simulink model "simActuatorPositionControl"  (R2022a)
settings: Solver=VariableStepAuto  StartTime=0.0  StopTime=10  FixedStep=0.001  MaxStep=0.01  RelTol=1e-3
InitFcn:
  | addpath('SCADA');
  | initFcn_SCADA;
model workspace (MAT data in the model file):
  WECmotionOnOff = Simulink.Parameter
  WECmotionOnOff.Value = 1
  WECmotionOnOff.DataType = 'auto'
  WECmotionOnOff.Complexity = 'real'
  WECmotionOnOff.Dimensions = [1 1]
values from neighbouring files (symbols this model uses):
  s = scatter(X(iVar),Y(iVar),100,[color(N-i+1,:)])    [postprocess_datafiles_accum_wRV.m]
undefined symbols (not defined in the file or in its folder): g, HIL_act_A_cap, HIL_act_A_rod, HIL_H1T_kd, HIL_H1T_ki, HIL_H1T_kp, HIL_H1T_P1fBias, HIL_H1T_P1negCutIn, HIL_H1T_P1posCutIn, HIL_H1T_P2fBias, HIL_H1T_P2negCutIn, HIL_H1T_P2posCutIn, HIL_scale_sys, HIL_WECpump_A_cap, HIL_WECpump_A_rod, HIL_WECpump_ang2lin, HIL_WECpump_negativeCtrlLimit, HIL_WECpump_negativeLimit, HIL_WECpump_positiveCtrlLimit, HIL_WECpump_positiveLimit, rho, wave_phi, wave_S_w, WEC_A_rad, WEC_B_rad, WEC_dw, WEC_F_amp, WEC_h, WEC_I, WEC_I_inf, WEC_ICs, WEC_L_cm, WEC_L_flap, WEC_m, WEC_phi_e, WEC_T, WEC_W, WEC_w
libraries: fl_lib x24, sh_lib x22, nesl_utility x11, slpidlib x1, simulink x1
(part 1 of 2)
settings Model: TunableVars=motionOnOff  TunableVarsStorageClass=ExportedGlobal  Creator=simmo536  LastModifiedBy=simmo536
settings SolverCC: ZeroCrossAlgorithm=Adaptive
settings OptimizationCC: DefaultParameterBehavior=Inlined
settings DebuggingCC: IgnoredZcDiagnostic=none
settings RTWCC: Toolchain=Microsoft Visual C++ 2019 v16.0 | nmake (64-bit Windows)

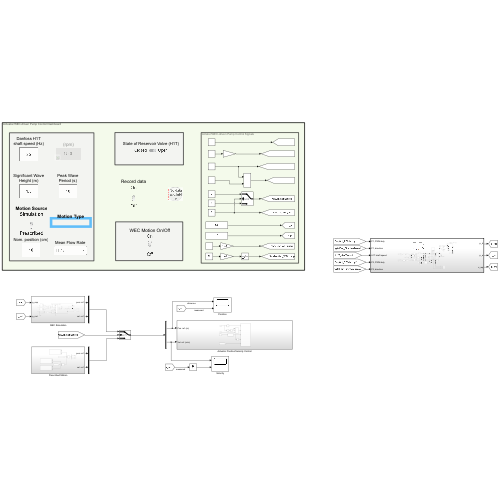
[thumbnail: Simulink's stored preview of the top-level diagram]
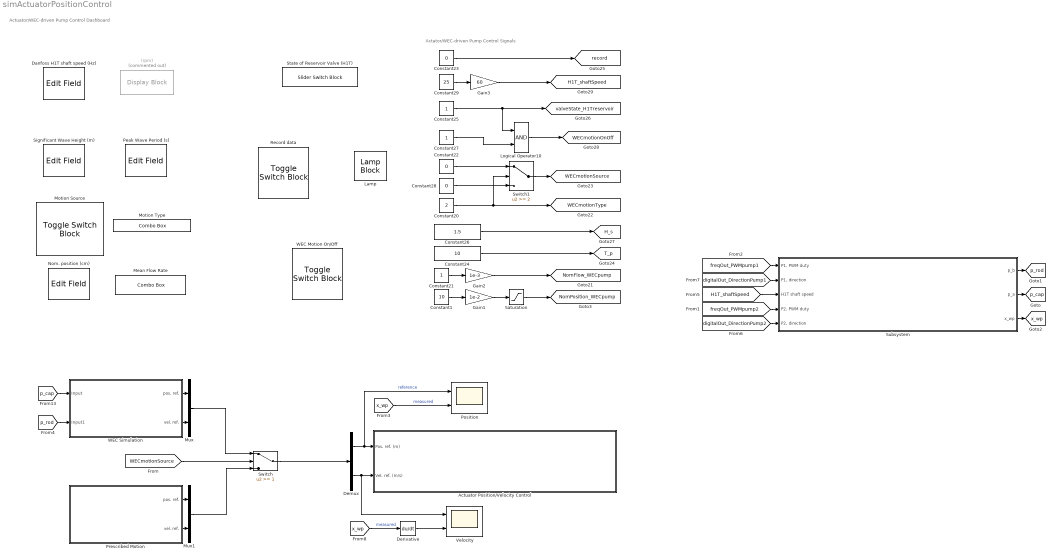
== system simActuatorPositionControl ==
  note: Actator/WEC-driven Pump Control Signals
  note: Actuator/WEC-driven Pump Control Dashboard
  (rpm) : DisplayBlock  Commented=on  LabelPosition=Hide  Format=long  Transparency=1
  Actuator Position/Velocity Control : Subsystem
  Constant1 : Constant  Value=10
  Constant20 : Constant  Value=2
  Constant21 : Constant
  Constant22 : Constant  Value=0
  Constant23 : Constant  Value=0
  Constant24 : Constant  Value=10
  Constant25 : Constant
  Constant26 : Constant  Value=1.5
  Constant27 : Constant
  Constant28 : Constant  Value=0
  Constant29 : Constant  Value=25
  Danfoss H1T shaft speed (Hz) : EditField  LabelPosition=Hide  ShowInitialText=on  Alignment=Center
  Demux : Demux  Outputs=2
  Derivative : Derivative
  Gain1 : Gain  Gain=1e-2
  Gain2 : Gain  Gain=1e-3
  Gain3 : Gain  Gain=60
  Lamp : LampBlock  LabelPosition=Hide
  Logical Operator10 : Logic  AllPortsSameDT=off  OutDataTypeStr=boolean
  Mean Flow Rate : ComboBox  LabelPosition=Hide  SelectedLabel=1 L/s
      settings: Values={{'0 L/s', '1 L/s', '2 L/2'}, [0 1 2]}
  Motion Source : ToggleSwitchBlock  LabelPosition=Hide
      settings: Values={{'Prescribed', 'Simulation'}, [0 1]}
  Motion Type : ComboBox  LabelPosition=Hide  SelectedLabel=Regular Waves
      settings: Values={{'Flow, Constant', 'Regular Waves', 'Irregular Waves', 'Position, Constant'}, [0 2 3 1]}
  Mux : Mux  Inputs=2
  Mux1 : Mux  Inputs=2
  Nom. position (cm) : EditField  LabelPosition=Hide  ShowInitialText=on  Alignment=Center
  Peak Wave Period (s) : EditField  LabelPosition=Hide  ShowInitialText=on  Alignment=Center
  Position : Scope  NumInputPorts=2
  Prescribed Motion : Subsystem
  Record data : ToggleSwitchBlock  LabelPosition=Hide
      settings: Values={{'Off', 'On'}, [0 1]}
  Saturation : Saturate
  Significant Wave Height (m) : EditField  LabelPosition=Hide  ShowInitialText=on  Alignment=Center
  State of Reservoir Valve (H1T) : SliderSwitchBlock  LabelPosition=Hide
      settings: Values={{'Closed', 'Open'}, [0 1]}
  Subsystem : Subsystem  TreatAsAtomicUnit=on
  Switch : Switch  Threshold=1  SaturateOnIntegerOverflow=off  InputSameDT=off
  Switch1 : Switch  Threshold=2  SaturateOnIntegerOverflow=off  InputSameDT=off
  Velocity : Scope  NumInputPorts=2
  WEC Motion On/Off : ToggleSwitchBlock  LabelPosition=Hide
      settings: Values={{'Off', 'On'}, [0 1]}
  WEC Simulation : Subsystem
  tag scope: H1T_shaftSpeed=global, H_s=global, NomFlow_WECpump=global, NomPosition_WECpump=global, T_p=global, WECmotionOnOff=global, WECmotionSource=global, WECmotionType=global, p_cap=global, p_rod=global, record=global, valveState_H1Treservoir=global, x_wp=global
  wires:
  [WECmotionSource] -> Switch/2
  Switch/1 -> Demux/1
  Demux/2 -> Velocity/1, Actuator Position/Velocity Control/2(Vel. ref. (m/s))
  Demux/1 -> Position/1, Actuator Position/Velocity Control/1(Pos. ref. (m))  "reference"
  Constant21/1 -> Gain2/1
  Constant29/1 -> Gain3/1
  Constant28/1 -> Switch1/3
  Gain3/1 -> [H1T_shaftSpeed]
  Switch1/1 -> [WECmotionSource]
  Constant20/1 -> Switch1/2, [WECmotionType]
  Logical Operator10/1 -> [WECmotionOnOff]
  Constant23/1 -> [record]
  Constant22/1 -> Switch1/1
  Constant25/1 -> Logical Operator10/1, [valveState_H1Treservoir]
  Constant26/1 -> [H_s]
  Constant24/1 -> [T_p]
  Gain2/1 -> [NomFlow_WECpump]
  [x_wp] -> Position/2  "measured"
  Constant27/1 -> Logical Operator10/2
  [p_cap] -> WEC Simulation/1(Input)
  WEC Simulation/1(pos. ref.) -> Mux/1
  [p_rod] -> WEC Simulation/2(Input1)
  WEC Simulation/2(vel. ref.) -> Mux/2
  Mux/1 -> Switch/1
  Prescribed Motion/2(vel. ref.) -> Mux1/2
  Mux1/1 -> Switch/3
  Prescribed Motion/1(pos. ref.) -> Mux1/1
  [freqOut_PWMpump1] -> Subsystem/1("P1, PWM duty")
  [digitalOut_DirectionPump1] -> Subsystem/2("P1, direction")
  [H1T_shaftSpeed] -> Subsystem/3(H1T shaft speed)
  [freqOut_PWMpump2] -> Subsystem/4("P2, PWM duty")
  [digitalOut_DirectionPump2] -> Subsystem/5("P2, direction")
  Subsystem/1(p_b) -> [p_rod]
  Subsystem/2(p_a) -> [p_cap]
  Subsystem/3(x_wp) -> [x_wp]
  Derivative/1 -> Velocity/2
  [x_wp] -> Derivative/1  "measured"
  Gain1/1 -> Saturation/1
  Constant1/1 -> Gain1/1
  Saturation/1 -> [NomPosition_WECpump]

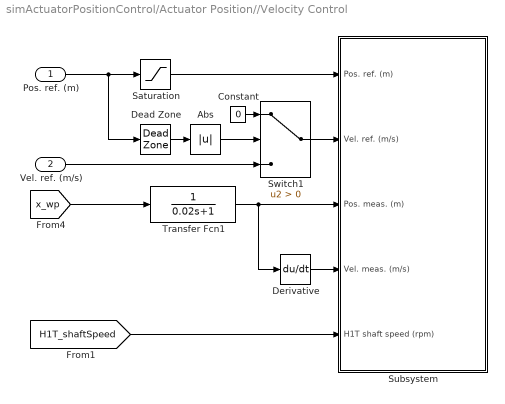
== system simActuatorPositionControl/Actuator Position//Velocity Control ==
  Pos. ref. (m) : Inport
  Vel. ref. (m/s) : Inport  Port=2
  Abs : Abs  SaturateOnIntegerOverflow=off
  Constant : Constant  Value=0
  Dead Zone : DeadZone  LowerValue=HIL_WECpump_negativeCtrlLimit  UpperValue=HIL_WECpump_positiveCtrlLimit
  Derivative : Derivative
  Saturation : Saturate  UpperLimit=HIL_WECpump_positiveCtrlLimit  LowerLimit=HIL_WECpump_negativeCtrlLimit
  Subsystem : Subsystem
  Switch1 : Switch  Criteria=u2 > Threshold  SaturateOnIntegerOverflow=off  InputSameDT=off
  Transfer Fcn1 : TransferFcn  Denominator=[0.02 1]
  wires:
  [x_wp] -> Transfer Fcn1/1
  Pos. ref. (m)/1 -> Saturation/1, Dead Zone/1
  Derivative/1 -> Subsystem/4(Vel. meas. (m/s))
  [H1T_shaftSpeed] -> Subsystem/5(H1T shaft speed (rpm))
  Transfer Fcn1/1 -> Subsystem/3(Pos. meas. (m)), Derivative/1
  Saturation/1 -> Subsystem/1(Pos. ref. (m))
  Dead Zone/1 -> Abs/1
  Abs/1 -> Switch1/2
  Constant/1 -> Switch1/1
  Switch1/1 -> Subsystem/2(Vel. ref. (m/s))
  Vel. ref. (m/s)/1 -> Switch1/3

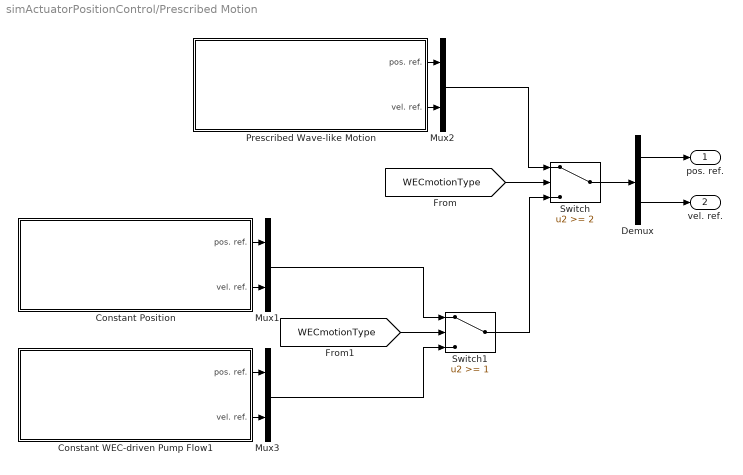
== system simActuatorPositionControl/Prescribed Motion ==
  Constant Position : Subsystem
  Constant WEC-driven Pump Flow1 : Subsystem
  Demux : Demux  Outputs=2
  Mux1 : Mux  Inputs=2
  Mux2 : Mux  Inputs=2
  Mux3 : Mux  Inputs=2
  Prescribed Wave-like Motion : Subsystem
  Switch : Switch  Threshold=2  SaturateOnIntegerOverflow=off  InputSameDT=off
  Switch1 : Switch  Threshold=1  SaturateOnIntegerOverflow=off  InputSameDT=off
  pos. ref. : Outport
  vel. ref. : Outport  Port=2
  wires:
  Prescribed Wave-like Motion/2(vel. ref.) -> Mux2/2
  Prescribed Wave-like Motion/1(pos. ref.) -> Mux2/1
  Mux2/1 -> Switch/1
  Demux/2 -> vel. ref./1
  Demux/1 -> pos. ref./1
  Constant Position/1(pos. ref.) -> Mux1/1
  Constant Position/2(vel. ref.) -> Mux1/2
  [WECmotionType] -> Switch/2
  Switch/1 -> Demux/1
  Constant WEC-driven Pump Flow1/2(vel. ref.) -> Mux3/2
  Constant WEC-driven Pump Flow1/1(pos. ref.) -> Mux3/1
  Mux3/1 -> Switch1/3
  [WECmotionType] -> Switch1/2
  Switch1/1 -> Switch/3
  Mux1/1 -> Switch1/1

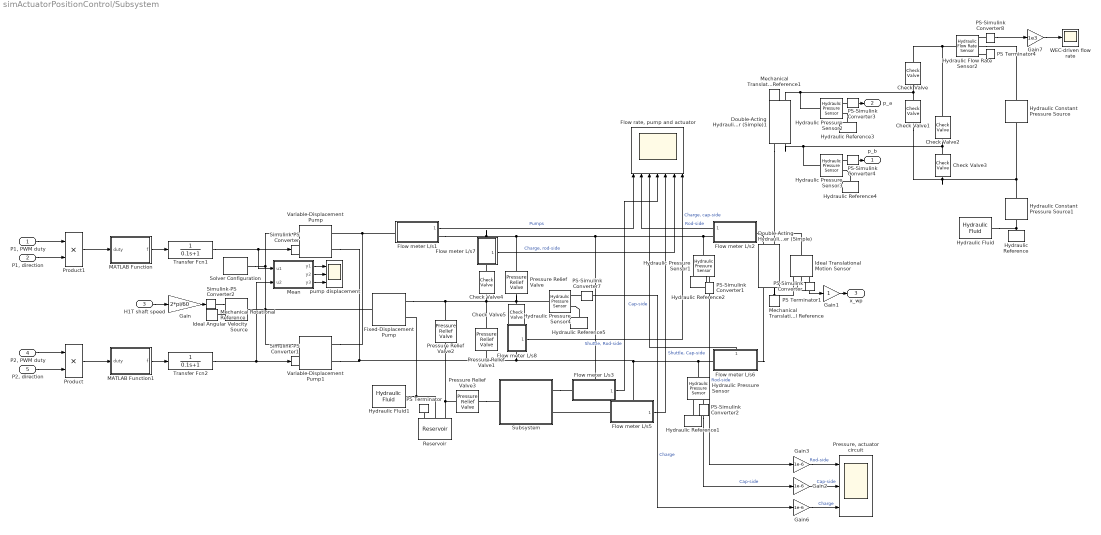
== system simActuatorPositionControl/Subsystem ==
  "P1, PWM duty" : Inport
  "P1, direction" : Inport  Port=2
  H1T shaft speed : Inport  Port=3
  "P2, PWM duty" : Inport  Port=4
  "P2, direction" : Inport  Port=5
  Check Valve{,1..3} (4 alike) : sh_lib/Valves/Directional Valves/Check Valve  area_max=6.1e-4 m^2  pres_crack=10 psi  pres_max=15 psi  C_d=0.7  A_leak=1e-12 m^2  lam_spec=1  B_lam=0.999  Re_cr=12  dynamic=0  tau=0.1 s  area_init=1e-12 m^2
      settings: SourceProductBaseCode=SH  InternalSimscapePortConfiguration="{\"Bottom\":[],\"Left\":[{\"id\":\"A\",\"label\":\"A\",\"type\":\"foundation.hydraulic.hydraulic\"}],\"Right\":[{\"id\":\"B\",\"label\":\"B\",\"type\":\"foundation.hydraulic.hydraulic\"}],\"Top\":[]}"
  Check Valve4 : sh_lib/Valves/Directional Valves/Check Valve  area_max=1e-4 m^2  pres_crack=5 bar  pres_max=6 bar  C_d=0.7  A_leak=1e-12 m^2  lam_spec=1  B_lam=0.999  Re_cr=12  dynamic=0  tau=0.1 s  area_init=1e-12 m^2
      settings: SourceProductBaseCode=SH  InternalSimscapePortConfiguration="{\"Bottom\":[],\"Left\":[{\"id\":\"A\",\"label\":\"A\",\"type\":\"foundation.hydraulic.hydraulic\"}],\"Right\":[{\"id\":\"B\",\"label\":\"B\",\"type\":\"foundation.hydraulic.hydraulic\"}],\"Top\":[]}"
  Check Valve5 : sh_lib/Valves/Directional Valves/Check Valve  area_max=1e-4 m^2  pres_crack=5 bar  pres_max=6 bar  C_d=0.7  A_leak=1e-12 m^2  lam_spec=1  B_lam=0.999  Re_cr=12  dynamic=0  tau=0.1 s  area_init=1e-12 m^2
      settings: SourceProductBaseCode=SH  InternalSimscapePortConfiguration="{\"Bottom\":[],\"Left\":[{\"id\":\"A\",\"label\":\"A\",\"type\":\"foundation.hydraulic.hydraulic\"}],\"Right\":[{\"id\":\"B\",\"label\":\"B\",\"type\":\"foundation.hydraulic.hydraulic\"}],\"Top\":[]}"
  Double-Acting Hydraulic Cylinder (Simple) : sh_lib/Hydraulic Cylinders/Double-Acting Hydraulic Cylinder (Simple)  area_A=HIL_act_A_cap m^2  area_B=HIL_act_A_rod m^2  stroke=1 m  init_pos=0.5 m  penetr_coeff=1e12 N*s/m^2  or=1
      settings: SourceProductBaseCode=SH  InternalSimscapePortConfiguration="{\"Bottom\":[],\"Left\":[{\"id\":\"C\",\"label\":\"C\",\"type\":\"foundation.mechanical.translational.translational\"},{\"id\":\"A\",\"label\":\"A\",\"type\":\"foundation.hydraulic.hydraulic\"}],\"Right\":[{\"id\":\"R\",\"label\":\"R\",\"type\":\"foundation.mechanical.translational.translational\"},{\"id\":\"B\",\"label\":\"B\",\"type\":\"foundation.hydraulic.hydraulic\"}],\"Top\":[]}"
  Double-Acting Hydraulic Cylinder (Simple)1 : sh_lib/Hydraulic Cylinders/Double-Acting Hydraulic Cylinder (Simple)  area_A=HIL_WECpump_A_cap m^2  area_B=HIL_WECpump_A_rod m^2  stroke=HIL_WECpump_positiveLimit - HIL_WECpump_negativeLimit m  init_pos=HIL_WECpump_positiveLimit m  penetr_coeff=1e12 N*s/m^2  or=1
      settings: SourceProductBaseCode=SH  InternalSimscapePortConfiguration="{\"Bottom\":[],\"Left\":[{\"id\":\"C\",\"label\":\"C\",\"type\":\"foundation.mechanical.translational.translational\"},{\"id\":\"A\",\"label\":\"A\",\"type\":\"foundation.hydraulic.hydraulic\"}],\"Right\":[{\"id\":\"R\",\"label\":\"R\",\"type\":\"foundation.mechanical.translational.translational\"},{\"id\":\"B\",\"label\":\"B\",\"type\":\"foundation.hydraulic.hydraulic\"}],\"Top\":[]}"
  Fixed-Displacement Pump : sh_lib/Pumps and Motors/Fixed-Displacement Pump  D=26.7 cm^3/rev  loss_spec=1  w_nominal=188 rad/s  pr_nominal=100e5 Pa  visc_nominal=18 cSt  dens_nominal=900 kg/m^3  efficiency_vol=0.92  no_load_torque=0.05 N*m  torque_pressure_coeff=0.6e-6 N*m/Pa  p_diff_eff_TLU=[100000, 1000000, 2000000] Pa  omega_eff_TLU=[25, 50, 100, 200, 300, 400] rad/s  vol_eff_TLU=[.816, .908, .954, .977, .981, .984; .325, .663, .831, .916, .925, .946; .137, .568, .78, .892, .893, .91]  mech_eff_TLU=[.996, .996, .996, .996, .996, .996; .988, .989, .989, .989, .989, .99; .981, .981, .982, .982, .983, .984]  p_diff_loss_TLU=[100000, 1000000, 2000000] Pa  omega_loss_TLU=[25, 50, 100, 200, 300, 400] rad/s  vol_loss_TLU=[.023, .023, .023, .023, .0285, .032; .0844, .0842, .0845, .084, .1125, .108; .1079, .108, .11, .108, .1605, .18] * 1e-3 m^3/s  mech_loss_TLU=[.002, .002, .002, .002, .002, .002; .0607, .0556, .0556, .0556, .0556, .0505; .1937, .1937, .1833, .1833, .1729, .1626] N*m  pressure_threshold=1e5 Pa  omega_threshold=10 rad/s  quadrant_check=0  pressure_check=0  min_valid_pressure=0 Pa  vol_eff_min=1e-3  vol_eff_max=1  mech_eff_min=1e-3  mech_eff_max=1
      settings: SourceProductBaseCode=SH  InternalSimscapePortConfiguration="{\"Bottom\":[],\"Left\":[{\"id\":\"S\",\"label\":\"S\",\"type\":\"foundation.mechanical.rotational.rotational\"}],\"Right\":[{\"id\":\"P\",\"label\":\"P\",\"type\":\"foundation.hydraulic.hydraulic\"},{\"id\":\"T\",\"label\":\"T\",\"type\":\"foundation.hydraulic.hydraulic\"}],\"Top\":[]}"
  Flow meter L/s{1..3,5..8} (7 alike) : Subsystem  ReferencedSubsystem=Flow_meter_L_s
      Flow meter L/s2 settings: PortSchema="{\"entries\":[{\"content\":{\"sides\":[{\"content\":{\"connectorIds\":[\"Out1\",\"LConn1\"]},\"type\":\"ConnectorPlacement.EquallySpacedRectSide\",\"uuid\":\"d44e5720-9e66-471e-94a4-9637237ee7d4\"},{\"content\":{\"connectorIds\":[\"RConn1\"],\"side\":\"RIGHT\"},\"type\":\"ConnectorPlacement.EquallySpacedRectSide\",\"uuid\":\"c0bd2997-7dbc-4043-b61a-302206a871bf\"},{\"content\":{\"connectorIds\":[],\"side\":\"TOP\"},\"type\":\"ConnectorPlacement.EquallySpacedRectSide\",\"uuid\":\"335e9987-789f-4915-b98a-4a003ac546c2\"}]},\"type\":\"ConnectorPlacement.EquallySpacedConnector\",\"uuid\":\"0505cca6-80c9-4470-9ce3-a34d7daa8e4f\"}],\"packageUris\":[\"http://schema.mathworks.com/mf0/Connector/R2020b\"],\"version\":\"1.0\"}"
      Flow meter L/s3 settings: PortSchema="{\"entries\":[{\"content\":{\"sides\":[{\"content\":{\"connectorIds\":[\"Out1\"]},\"type\":\"ConnectorPlacement.EquallySpacedRectSide\",\"uuid\":\"d44e5720-9e66-471e-94a4-9637237ee7d4\"},{\"content\":{\"connectorIds\":[\"RConn1\"],\"side\":\"RIGHT\"},\"type\":\"ConnectorPlacement.EquallySpacedRectSide\",\"uuid\":\"c0bd2997-7dbc-4043-b61a-302206a871bf\"},{\"content\":{\"connectorIds\":[\"LConn1\"],\"side\":\"TOP\"},\"type\":\"ConnectorPlacement.EquallySpacedRectSide\",\"uuid\":\"335e9987-789f-4915-b98a-4a003ac546c2\"}]},\"type\":\"ConnectorPlacement.EquallySpacedConnector\",\"uuid\":\"0505cca6-80c9-4470-9ce3-a34d7daa8e4f\"}],\"packageUris\":[\"http://schema.mathworks.com/mf0/Connector/R2020b\"],\"version\":\"1.0\"}"
      Flow meter L/s5 settings: PortSchema="{\"entries\":[{\"content\":{\"sides\":[{\"content\":{\"connectorIds\":[\"Out1\"]},\"type\":\"ConnectorPlacement.EquallySpacedRectSide\",\"uuid\":\"d44e5720-9e66-471e-94a4-9637237ee7d4\"},{\"content\":{\"connectorIds\":[\"RConn1\"],\"side\":\"RIGHT\"},\"type\":\"ConnectorPlacement.EquallySpacedRectSide\",\"uuid\":\"c0bd2997-7dbc-4043-b61a-302206a871bf\"},{\"content\":{\"connectorIds\":[\"LConn1\"],\"side\":\"TOP\"},\"type\":\"ConnectorPlacement.EquallySpacedRectSide\",\"uuid\":\"335e9987-789f-4915-b98a-4a003ac546c2\"}]},\"type\":\"ConnectorPlacement.EquallySpacedConnector\",\"uuid\":\"0505cca6-80c9-4470-9ce3-a34d7daa8e4f\"}],\"packageUris\":[\"http://schema.mathworks.com/mf0/Connector/R2020b\"],\"version\":\"1.0\"}"
      Flow meter L/s6 settings: PortSchema="{\"entries\":[{\"content\":{\"sides\":[{\"content\":{\"connectorIds\":[\"LConn1\"]},\"type\":\"ConnectorPlacement.EquallySpacedRectSide\",\"uuid\":\"d44e5720-9e66-471e-94a4-9637237ee7d4\"},{\"content\":{\"connectorIds\":[\"RConn1\"],\"side\":\"RIGHT\"},\"type\":\"ConnectorPlacement.EquallySpacedRectSide\",\"uuid\":\"c0bd2997-7dbc-4043-b61a-302206a871bf\"},{\"content\":{\"connectorIds\":[\"Out1\"],\"side\":\"TOP\"},\"type\":\"ConnectorPlacement.EquallySpacedRectSide\",\"uuid\":\"335e9987-789f-4915-b98a-4a003ac546c2\"},{\"content\":{\"connectorIds\":[],\"side\":\"BOTTOM\"},\"type\":\"ConnectorPlacement.EquallySpacedRectSide\",\"uuid\":\"a3edc401-22a1-4880-a190-f88c0fe4af5a\"}]},\"type\":\"ConnectorPlacement.EquallySpacedConnector\",\"uuid\":\"0505cca6-80c9-4470-9ce3-a34d7daa8e4f\"}],\"packageUris\":[\"http://schema.mathworks.com/mf0/Connector/R2020b\"],\"version\":\"1.0\"}"
      Flow meter L/s7 settings: PortSchema="{\"entries\":[{\"content\":{\"sides\":[{\"content\":{\"connectorIds\":[\"LConn1\"]},\"type\":\"ConnectorPlacement.EquallySpacedRectSide\",\"uuid\":\"d44e5720-9e66-471e-94a4-9637237ee7d4\"},{\"content\":{\"connectorIds\":[\"RConn1\"],\"side\":\"RIGHT\"},\"type\":\"ConnectorPlacement.EquallySpacedRectSide\",\"uuid\":\"c0bd2997-7dbc-4043-b61a-302206a871bf\"},{\"content\":{\"connectorIds\":[],\"side\":\"TOP\"},\"type\":\"ConnectorPlacement.EquallySpacedRectSide\",\"uuid\":\"335e9987-789f-4915-b98a-4a003ac546c2\"},{\"content\":{\"connectorIds\":[\"Out1\"],\"side\":\"BOTTOM\"},\"type\":\"ConnectorPlacement.EquallySpacedRectSide\",\"uuid\":\"a3edc401-22a1-4880-a190-f88c0fe4af5a\"}]},\"type\":\"ConnectorPlacement.EquallySpacedConnector\",\"uuid\":\"0505cca6-80c9-4470-9ce3-a34d7daa8e4f\"}],\"packageUris\":[\"http://schema.mathworks.com/mf0/Connector/R2020b\"],\"version\":\"1.0\"}"
      Flow meter L/s8 settings: PortSchema="{\"entries\":[{\"content\":{\"sides\":[{\"content\":{\"connectorIds\":[\"LConn1\"]},\"type\":\"ConnectorPlacement.EquallySpacedRectSide\",\"uuid\":\"d44e5720-9e66-471e-94a4-9637237ee7d4\"},{\"content\":{\"connectorIds\":[\"RConn1\"],\"side\":\"RIGHT\"},\"type\":\"ConnectorPlacement.EquallySpacedRectSide\",\"uuid\":\"c0bd2997-7dbc-4043-b61a-302206a871bf\"},{\"content\":{\"connectorIds\":[\"Out1\"],\"side\":\"TOP\"},\"type\":\"ConnectorPlacement.EquallySpacedRectSide\",\"uuid\":\"335e9987-789f-4915-b98a-4a003ac546c2\"},{\"content\":{\"connectorIds\":[],\"side\":\"BOTTOM\"},\"type\":\"ConnectorPlacement.EquallySpacedRectSide\",\"uuid\":\"a3edc401-22a1-4880-a190-f88c0fe4af5a\"}]},\"type\":\"ConnectorPlacement.EquallySpacedConnector\",\"uuid\":\"0505cca6-80c9-4470-9ce3-a34d7daa8e4f\"}],\"packageUris\":[\"http://schema.mathworks.com/mf0/Connector/R2020b\"],\"version\":\"1.0\"}"
  "Flow rate, pump and actuator" : Scope  NumInputPorts=7
  Gain : Gain  Gain=2*pi/60
  Gain1 : Gain
  Gain2 : Gain  Gain=1e-6
  Gain3 : Gain  Gain=1e-6
  Gain6 : Gain  Gain=1e-6
  Gain7 : Gain  Gain=1e3
  Hydraulic Constant Pressure Source : fl_lib/Hydraulic/Hydraulic Sources/Hydraulic Constant Pressure Source  commanded_pressure=6 MPa
      settings: SourceProductBaseCode=PW,SS,VE  InternalSimscapePortConfiguration="{\"Bottom\":[],\"Left\":[{\"id\":\"P\",\"label\":\"P\",\"type\":\"foundation.hydraulic.hydraulic\"}],\"Right\":[{\"id\":\"T\",\"label\":\"T\",\"type\":\"foundation.hydraulic.hydraulic\"}],\"Top\":[]}"
  Hydraulic Constant Pressure Source1 : fl_lib/Hydraulic/Hydraulic Sources/Hydraulic Constant Pressure Source  commanded_pressure=0.5 MPa
      settings: SourceProductBaseCode=PW,SS,VE  InternalSimscapePortConfiguration="{\"Bottom\":[],\"Left\":[{\"id\":\"P\",\"label\":\"P\",\"type\":\"foundation.hydraulic.hydraulic\"}],\"Right\":[{\"id\":\"T\",\"label\":\"T\",\"type\":\"foundation.hydraulic.hydraulic\"}],\"Top\":[]}"
  Hydraulic Flow Rate Sensor2 : fl_lib/Hydraulic/Hydraulic Sensors/Hydraulic Flow Rate Sensor
      settings: SourceProductBaseCode=PW,SS,VE
  Hydraulic Fluid : sh_lib/Hydraulic Utilities/Hydraulic Fluid  SelFluid=24  SysTemp=60  TrapAir=0.005  ViscDerFactor=1  range_error=2
  Hydraulic Fluid1 : sh_lib/Hydraulic Utilities/Hydraulic Fluid  SelFluid=15  SysTemp=60  TrapAir=0.001  ViscDerFactor=1  range_error=2
  Hydraulic Pressure Sensor{,1..4} (5 alike) : fl_lib/Hydraulic/Hydraulic Sensors/Hydraulic Pressure Sensor
      settings: SourceProductBaseCode=PW,SS,VE
  Hydraulic Reference{,1..5} (6 alike) : fl_lib/Hydraulic/Hydraulic Elements/Hydraulic Reference
      settings: SourceProductBaseCode=PW,SS,VE
  Ideal Angular Velocity Source : fl_lib/Mechanical/Mechanical Sources/Ideal Angular Velocity Source
      settings: SourceProductBaseCode=PW,SS,VE
  Ideal Translational Motion Sensor : fl_lib/Mechanical/Mechanical Sensors/Ideal Translational Motion Sensor  offset=0 m
      settings: SourceProductBaseCode=PW,SS,VE
  MATLAB Function : MATLAB Function  TreatAsAtomicUnit=on
  MATLAB Function1 : MATLAB Function  TreatAsAtomicUnit=on
  Mean : MATLAB Function  TreatAsAtomicUnit=on
  Mechanical Rotational Reference : fl_lib/Mechanical/Rotational Elements/Mechanical Rotational Reference
      settings: SourceProductBaseCode=PW,SS,VE
  Mechanical Translational Reference : fl_lib/Mechanical/Translational Elements/Mechanical Translational Reference
      settings: SourceProductBaseCode=PW,SS,VE
  Mechanical Translational Reference1 : fl_lib/Mechanical/Translational Elements/Mechanical Translational Reference
      settings: SourceProductBaseCode=PW,SS,VE
  PS Terminator : fl_lib/Physical Signals/Sinks/PS Terminator
      settings: SourceProductBaseCode=PW,SS,VE
  PS Terminator1 : fl_lib/Physical Signals/Sinks/PS Terminator
      settings: SourceProductBaseCode=PW,SS,VE
  PS Terminator4 : fl_lib/Physical Signals/Sinks/PS Terminator
      settings: SourceProductBaseCode=PW,SS,VE
  PS-Simulink Converter{,3..4,8} (4 alike) : nesl_utility/PS-Simulink Converter  PhysicalDomain=network_engine_domain  SubClassName=ps_output  LeftPortType=input  RightPortType=output  PseudoPeriodic=off  Frequencies=[]  VectorFormat=1-D array  Unit=inherit  AffineConversion=off
      settings: SourceProductBaseCode=SS,PW,VE
  PS-Simulink Converter1 : nesl_utility/PS-Simulink Converter  PhysicalDomain=network_engine_domain  SubClassName=ps_output  LeftPortType=input  RightPortType=output  PseudoPeriodic=off  Frequencies=[]  VectorFormat=1-D array  Unit=Pa  AffineConversion=off
      settings: SourceProductBaseCode=SS,PW,VE
  PS-Simulink Converter2 : nesl_utility/PS-Simulink Converter  PhysicalDomain=network_engine_domain  SubClassName=ps_output  LeftPortType=input  RightPortType=output  PseudoPeriodic=off  Frequencies=[]  VectorFormat=1-D array  Unit=Pa  AffineConversion=off
      settings: SourceProductBaseCode=SS,PW,VE
  PS-Simulink Converter7 : nesl_utility/PS-Simulink Converter  PhysicalDomain=network_engine_domain  SubClassName=ps_output  LeftPortType=input  RightPortType=output  PseudoPeriodic=off  Frequencies=[]  VectorFormat=1-D array  Unit=Pa  AffineConversion=off
      settings: SourceProductBaseCode=SS,PW,VE
  Pressure Relief Valve : sh_lib/Valves/Pressure Control Valves/Pressure Relief Valve  valve_area_spec=1  p_diff_TLU=[30.15e5 : 15e3 : 31.35e5] Pa  area_TLU=[1 : 1 : 9] .* 1e-5 m^2  area_max=1e-4 m^2  pres_set=20 MPa  reg_range=5e5 Pa  C_d=0.7  A_leak=1e-12 m^2  lam_spec=1  B_lam=0.999  Re_cr=12  dynamic=0  tau=0.1 s  area_init=1e-12 m^2
      settings: SourceProductBaseCode=SH  InternalSimscapePortConfiguration="{\"Bottom\":[],\"Left\":[{\"id\":\"A\",\"label\":\"A\",\"type\":\"foundation.hydraulic.hydraulic\"}],\"Right\":[{\"id\":\"B\",\"label\":\"B\",\"type\":\"foundation.hydraulic.hydraulic\"}],\"Top\":[]}"
  Pressure Relief Valve1 : sh_lib/Valves/Pressure Control Valves/Pressure Relief Valve  valve_area_spec=1  p_diff_TLU=[30.15e5 : 15e3 : 31.35e5] Pa  area_TLU=[1 : 1 : 9] .* 1e-5 m^2  area_max=1e-4 m^2  pres_set=20 MPa  reg_range=5e5 MPa  C_d=0.7  A_leak=1e-12 m^2  lam_spec=1  B_lam=0.999  Re_cr=12  dynamic=0  tau=0.1 s  area_init=1e-12 m^2
      settings: SourceProductBaseCode=SH  InternalSimscapePortConfiguration="{\"Bottom\":[],\"Left\":[{\"id\":\"A\",\"label\":\"A\",\"type\":\"foundation.hydraulic.hydraulic\"}],\"Right\":[{\"id\":\"B\",\"label\":\"B\",\"type\":\"foundation.hydraulic.hydraulic\"}],\"Top\":[]}"
  Pressure Relief Valve2 : sh_lib/Valves/Pressure Control Valves/Pressure Relief Valve  valve_area_spec=1  p_diff_TLU=[30.15e5 : 15e3 : 31.35e5] Pa  area_TLU=[1 : 1 : 9] .* 1e-5 m^2  area_max=1e-4 m^2  pres_set=45 bar  reg_range=5e5 Pa  C_d=0.7  A_leak=1e-12 m^2  lam_spec=1  B_lam=0.999  Re_cr=12  dynamic=0  tau=0.1 s  area_init=1e-12 m^2
      settings: SourceProductBaseCode=SH  InternalSimscapePortConfiguration="{\"Bottom\":[],\"Left\":[{\"id\":\"A\",\"label\":\"A\",\"type\":\"foundation.hydraulic.hydraulic\"}],\"Right\":[{\"id\":\"B\",\"label\":\"B\",\"type\":\"foundation.hydraulic.hydraulic\"}],\"Top\":[]}"
  Pressure Relief Valve3 : sh_lib/Valves/Pressure Control Valves/Pressure Relief Valve  valve_area_spec=1  p_diff_TLU=[30.15e5 : 15e3 : 31.35e5] Pa  area_TLU=[1 : 1 : 9] .* 1e-5 m^2  area_max=1e-4 m^2  pres_set=40 bar  reg_range=5e5 Pa  C_d=0.7  A_leak=1e-12 m^2  lam_spec=1  B_lam=0.999  Re_cr=12  dynamic=0  tau=0.1 s  area_init=1e-12 m^2
      settings: SourceProductBaseCode=SH  InternalSimscapePortConfiguration="{\"Bottom\":[],\"Left\":[{\"id\":\"A\",\"label\":\"A\",\"type\":\"foundation.hydraulic.hydraulic\"}],\"Right\":[{\"id\":\"B\",\"label\":\"B\",\"type\":\"foundation.hydraulic.hydraulic\"}],\"Top\":[]}"
  "Pressure, actuator circuit" : Scope  NumInputPorts=3
  Product : Product
  Product1 : Product
  Reservoir : sh_lib/Hydraulic Utilities/Reservoir  press=0 Pa  init_volume=0.02 m^3  ret_diam=0.02 m  loss_coeff=1
      settings: SourceProductBaseCode=SH  InternalSimscapePortConfiguration="{\"Bottom\":[],\"Left\":[{\"id\":\"V\",\"label\":\"V\",\"type\":\"output\"},{\"id\":\"P\",\"label\":\"P\",\"type\":\"foundation.hydraulic.hydraulic\"},{\"id\":\"R\",\"label\":\"R\",\"type\":\"foundation.hydraulic.hydraulic\"}],\"Right\":[],\"Top\":[]}"
  Simulink-PS Converter : nesl_utility/Simulink-PS Converter  PhysicalDomain=network_engine_domain  SubClassName=ps_input  LeftPortType=input  RightPortType=output  PseudoPeriodic=off  Frequencies=[]  NoiseDistribution=none  NoiseParameters=[]  Unit=cm  AffineConversion=off  FilteringAndDerivatives=provide  SimscapeFilterOrder=1  InputFilterTimeConstant=0.001  UdotUserProvided=0
      settings: SourceProductBaseCode=SS,PW,VE
  Simulink-PS Converter1 : nesl_utility/Simulink-PS Converter  PhysicalDomain=network_engine_domain  SubClassName=ps_input  LeftPortType=input  RightPortType=output  PseudoPeriodic=off  Frequencies=[]  NoiseDistribution=none  NoiseParameters=[]  Unit=cm  AffineConversion=off  FilteringAndDerivatives=provide  SimscapeFilterOrder=1  InputFilterTimeConstant=0.001  UdotUserProvided=0
      settings: SourceProductBaseCode=SS,PW,VE
  Simulink-PS Converter2 : nesl_utility/Simulink-PS Converter  PhysicalDomain=network_engine_domain  SubClassName=ps_input  LeftPortType=input  RightPortType=output  PseudoPeriodic=off  Frequencies=[]  NoiseDistribution=none  NoiseParameters=[]  Unit=1  AffineConversion=off  FilteringAndDerivatives=provide  SimscapeFilterOrder=1  InputFilterTimeConstant=0.001  UdotUserProvided=0
      settings: SourceProductBaseCode=SS,PW,VE
  Solver Configuration : nesl_utility/Solver Configuration  PhysicalDomain=network_engine_domain  SubClassName=solver  LeftPortType=input  RightPortType=generic  Tones=[]  Harmonics=[]  SimulateNoise=off  Profile=off  UseLocalSampling=off  EnableSwitchedLinearOptims=on  FrequencyDomain=off  UseCCode=off  RelTol=0.001  AbsTol=1e-06  MinStep=1e-09  ToWorkspace=off  RevertToSquareIcSolve=off  NumHomotopyIterations=100  PhasorMode=off  PhasorModeNumHarmonics=1  IndexReductionMethod=DerivativeReplacement  DoDC=off  ResidualTolerance=1e-09  UseLocalSolver=off  LocalSolverChoice=NE_BACKWARD_EULER_ADVANCER  LocalSolverSampleTime=0.001  DoFixedCost=off  MaxNonlinIter=3  MaxModeIter=2  ComputeImpulses=off  ImpulseIterations=2  LinearAlgebra=auto  LinearAlgebraNumThread=0  EquationFormulation=NE_TIME_EF  DelaysMemoryBudget=1024  AutomaticFiltering=on  FilteringTimeConstant=0.001  PartitionStorageMethod=AS_NEEDED  PartitionMemoryBudget=1024  PartitionMethod=ROBUST
      settings: SourceProductBaseCode=SS,PW,VE
  Subsystem : Subsystem
  Transfer Fcn1 : TransferFcn  Denominator=[0.1 1]
  Transfer Fcn2 : TransferFcn  Denominator=[0.1 1]
  Variable-Displacement Pump : sh_lib/Pumps and Motors/Variable-Displacement Pump  mdl_type=1  stroke_max=1 cm  D_max=53.8 cm^3/rev  cntrl_mem_tab=[-.0075, -.0025, 0, .0025, .0075] m  displ_tab=[-30, -19, 0, 19, 30] cm^3/rev  interp_method=1  extrap_method=1  loss_spec=1  w_nominal=188 rad/s  pr_nominal=100e5 Pa  visc_nominal=18 cSt  dens_nominal=900 kg/m^3  efficiency_vol=0.92  no_load_torque=0.05 N*m  torque_pressure_coeff=0.6e-6 N*m/Pa  p_diff_eff_TLU=[100000, 1000000, 2000000] Pa  omega_eff_TLU=[25, 50, 100, 200, 300, 400] rad/s  displacement_eff_TLU=[-30, -19, 19, 30] cm^3/rev  vol_eff_TLU=repmat([.816, .908, .954, .977, .981, .984; .325, .663, .831, .916, .925, .946; .137, .568, .78, .892, .893, .91], 1, 1, 4)  mech_eff_TLU=repmat([.996, .996, .996, .996, .996, .996; .988, .989, .989, .989, .989, .99; .981, .981, .982, .982, .983, .984], 1, 1, 4)  p_diff_loss_TLU=[100000, 1000000, 2000000] Pa  omega_loss_TLU=[25, 50, 100, 200, 300, 400] rad/s  displacement_loss_TLU=[-30, -19, 19, 30] cm^3/rev  vol_loss_TLU=repmat([.023, .023, .023, .023, .0285, .032; .0844, .0842, .0845, .084, .1125, .108; .1079, .108, .11, .108, .1605, .18] * 1e-3, 1, 1, 4) m^3/s  mech_loss_TLU=repmat([.002, .002, .002, .002, .002, .002; .0607, .0556, .0556, .0556, .0556, .0505; .1937, .1937, .1833, .1833, .1729, .1626], 1, 1, 4) N*m  pressure_threshold=1e5 Pa  omega_threshold=10 rad/s  displacement_threshold=0.5 cm^3/rev  octant_check=0  pressure_check=0  min_valid_pressure=0 Pa  vol_eff_min=1e-3  vol_eff_max=1  mech_eff_min=1e-3  mech_eff_max=1
      settings: SourceProductBaseCode=SH  InternalSimscapePortConfiguration="{\"Bottom\":[],\"Left\":[{\"id\":\"C\",\"label\":\"C\",\"type\":\"input\"},{\"id\":\"S\",\"label\":\"S\",\"type\":\"foundation.mechanical.rotational.rotational\"}],\"Right\":[{\"id\":\"P\",\"label\":\"P\",\"type\":\"foundation.hydraulic.hydraulic\"},{\"id\":\"T\",\"label\":\"T\",\"type\":\"foundation.hydraulic.hydraulic\"}],\"Top\":[]}"
  Variable-Displacement Pump1 : sh_lib/Pumps and Motors/Variable-Displacement Pump  mdl_type=1  stroke_max=1 cm  D_max=53.8 cm^3/rev  cntrl_mem_tab=[-.0075, -.0025, 0, .0025, .0075] m  displ_tab=[-30, -19, 0, 19, 30] cm^3/rev  interp_method=1  extrap_method=1  loss_spec=1  w_nominal=188 rad/s  pr_nominal=100e5 Pa  visc_nominal=18 cSt  dens_nominal=900 kg/m^3  efficiency_vol=0.92  no_load_torque=0.05 N*m  torque_pressure_coeff=0.6e-6 N*m/Pa  p_diff_eff_TLU=[100000, 1000000, 2000000] Pa  omega_eff_TLU=[25, 50, 100, 200, 300, 400] rad/s  displacement_eff_TLU=[-30, -19, 19, 30] cm^3/rev  vol_eff_TLU=repmat([.816, .908, .954, .977, .981, .984; .325, .663, .831, .916, .925, .946; .137, .568, .78, .892, .893, .91], 1, 1, 4)  mech_eff_TLU=repmat([.996, .996, .996, .996, .996, .996; .988, .989, .989, .989, .989, .99; .981, .981, .982, .982, .983, .984], 1, 1, 4)  p_diff_loss_TLU=[100000, 1000000, 2000000] Pa  omega_loss_TLU=[25, 50, 100, 200, 300, 400] rad/s  displacement_loss_TLU=[-30, -19, 19, 30] cm^3/rev  vol_loss_TLU=repmat([.023, .023, .023, .023, .0285, .032; .0844, .0842, .0845, .084, .1125, .108; .1079, .108, .11, .108, .1605, .18] * 1e-3, 1, 1, 4) m^3/s  mech_loss_TLU=repmat([.002, .002, .002, .002, .002, .002; .0607, .0556, .0556, .0556, .0556, .0505; .1937, .1937, .1833, .1833, .1729, .1626], 1, 1, 4) N*m  pressure_threshold=1e5 Pa  omega_threshold=10 rad/s  displacement_threshold=0.5 cm^3/rev  octant_check=0  pressure_check=0  min_valid_pressure=0 Pa  vol_eff_min=1e-3  vol_eff_max=1  mech_eff_min=1e-3  mech_eff_max=1
      settings: SourceProductBaseCode=SH  InternalSimscapePortConfiguration="{\"Bottom\":[],\"Left\":[{\"id\":\"C\",\"label\":\"C\",\"type\":\"input\"},{\"id\":\"S\",\"label\":\"S\",\"type\":\"foundation.mechanical.rotational.rotational\"}],\"Right\":[{\"id\":\"P\",\"label\":\"P\",\"type\":\"foundation.hydraulic.hydraulic\"},{\"id\":\"T\",\"label\":\"T\",\"type\":\"foundation.hydraulic.hydraulic\"}],\"Top\":[]}"
  WEC-driven flow rate : Scope
  pump displacement : Scope  NumInputPorts=3
  p_b : Outport
  p_a : Outport  Port=2
  x_wp : Outport  Port=3
  wires:
  MATLAB Function/1(f) -> Transfer Fcn1/1
  "P2, direction"/1 -> Product/2
  Transfer Fcn2/1 -> Mean/2(u2), Simulink-PS Converter1/1
  Flow meter L/s2/1 -> "Flow rate, pump and actuator"/2  "Rod-side"
  Product/1 -> MATLAB Function1/1(duty)
  PS-Simulink Converter3/1 -> p_a/1
  PS-Simulink Converter/1 -> Gain1/1
  Gain3/1 -> "Pressure, actuator circuit"/1  "Rod-side"
  Gain2/1 -> "Pressure, actuator circuit"/2  "Cap-side"
  "P2, PWM duty"/1 -> Product/1
  Gain/1 -> Simulink-PS Converter2/1
  "P1, direction"/1 -> Product1/2
  Gain1/1 -> x_wp/1
  Flow meter L/s1/1 -> "Flow rate, pump and actuator"/1  "Pumps"
  PS-Simulink Converter4/1 -> p_b/1
  H1T shaft speed/1 -> Gain/1
  "P1, PWM duty"/1 -> Product1/1
  PS-Simulink Converter2/1 -> Gain2/1  "Cap-side"
  PS-Simulink Converter1/1 -> Gain3/1  "Rod-side"
  PS-Simulink Converter7/1 -> Gain6/1  "Charge"
  Gain6/1 -> "Pressure, actuator circuit"/3  "Charge"
  PS-Simulink Converter8/1 -> Gain7/1
  Gain7/1 -> WEC-driven flow rate/1
  MATLAB Function1/1(f) -> Transfer Fcn2/1
  Transfer Fcn1/1 -> Mean/1(u1), Simulink-PS Converter/1
  Product1/1 -> MATLAB Function/1(duty)
  Mean/1(y1) -> pump displacement/1
  Mean/3(y3) -> pump displacement/3
  Mean/2(y2) -> pump displacement/2
  Flow meter L/s3/1 -> "Flow rate, pump and actuator"/4  "Shuttle, Rod-side"
  Flow meter L/s5/1 -> "Flow rate, pump and actuator"/5  "Shuttle, Cap-side"
  Flow meter L/s6/1 -> "Flow rate, pump and actuator"/3  "Cap-side"
  Flow meter L/s7/1 -> "Flow rate, pump and actuator"/6  "Charge, rod-side"
  Flow meter L/s8/1 -> "Flow rate, pump and actuator"/7  "Charge, cap-side"
  connections:
  Mechanical Translational Reference/LConn1 -- Ideal Translational Motion Sensor/RConn1 -- Double-Acting Hydraulic Cylinder (Simple)/LConn1
  Check Valve4/LConn1 -- Pressure Relief Valve1/RConn1 -- Pressure Relief Valve/RConn1 -- Check Valve5/LConn1 -- Hydraulic Pressure Sensor4/LConn1 -- Pressure Relief Valve2/LConn1 -- Fixed-Displacement Pump/RConn1
  Double-Acting Hydraulic Cylinder (Simple)1/RConn1 -- Ideal Translational Motion Sensor/LConn1 -- Double-Acting Hydraulic Cylinder (Simple)/RConn1
  Check Valve/RConn1 -- Check Valve2/RConn1 -- Hydraulic Flow Rate Sensor2/LConn1
  Check Valve3/LConn1 -- Check Valve1/LConn1 -- Hydraulic Constant Pressure Source1/LConn1 -- Hydraulic Constant Pressure Source/RConn1
  Variable-Displacement Pump/LConn2 -- Variable-Displacement Pump1/LConn2 -- Ideal Angular Velocity Source/LConn1 -- Fixed-Displacement Pump/LConn1 -- Solver Configuration/RConn1
  Hydraulic Reference1/LConn1 -- Hydraulic Pressure Sensor/RConn1
  Hydraulic Reference2/LConn1 -- Hydraulic Pressure Sensor1/RConn1
  Hydraulic Constant Pressure Source1/RConn1 -- Hydraulic Reference/LConn1 -- Hydraulic Fluid/RConn1
  Pressure Relief Valve1/LConn1 -- Flow meter L/s6/LConn1 -- Hydraulic Pressure Sensor/LConn1 -- Flow meter L/s5/LConn1 -- Flow meter L/s8/RConn1 -- Variable-Displacement Pump/RConn1 -- Variable-Displacement Pump1/RConn1
  Double-Acting Hydraulic Cylinder (Simple)1/LConn2 -- Hydraulic Pressure Sensor2/LConn1 -- Check Valve1/RConn1 -- Check Valve/LConn1
  Ideal Translational Motion Sensor/RConn2 -- PS Terminator1/LConn1
  PS-Simulink Converter2/LConn1 -- Hydraulic Pressure Sensor/RConn2
  PS-Simulink Converter1/LConn1 -- Hydraulic Pressure Sensor1/RConn2
  Mechanical Rotational Reference/LConn1 -- Ideal Angular Velocity Source/RConn2
  Simulink-PS Converter1/RConn1 -- Variable-Displacement Pump1/LConn1
  Reservoir/LConn2 -- Hydraulic Fluid1/RConn1 -- Fixed-Displacement Pump/RConn2
  PS-Simulink Converter4/LConn1 -- Hydraulic Pressure Sensor3/RConn2
  Hydraulic Reference4/LConn1 -- Hydraulic Pressure Sensor3/RConn1
  Reservoir/LConn3 -- Pressure Relief Valve3/RConn1 -- Pressure Relief Valve2/RConn1
  Mechanical Translational Reference1/LConn1 -- Double-Acting Hydraulic Cylinder (Simple)1/LConn1
  Simulink-PS Converter/RConn1 -- Variable-Displacement Pump/LConn1
  Simulink-PS Converter2/RConn1 -- Ideal Angular Velocity Source/RConn1
  Reservoir/LConn1 -- PS Terminator/LConn1
  Double-Acting Hydraulic Cylinder (Simple)/RConn2 -- Flow meter L/s2/RConn1
  PS-Simulink Converter3/LConn1 -- Hydraulic Pressure Sensor2/RConn2
  Double-Acting Hydraulic Cylinder (Simple)1/RConn2 -- Hydraulic Pressure Sensor3/LConn1 -- Check Valve3/RConn1 -- Check Valve2/LConn1
  Hydraulic Reference3/LConn1 -- Hydraulic Pressure Sensor2/RConn1
  PS-Simulink Converter/LConn1 -- Ideal Translational Motion Sensor/RConn3
  Hydraulic Reference5/LConn1 -- Hydraulic Pressure Sensor4/RConn1
  PS-Simulink Converter7/LConn1 -- Hydraulic Pressure Sensor4/RConn2
  Variable-Displacement Pump1/RConn2 -- Variable-Displacement Pump/RConn2 -- Flow meter L/s1/LConn1
  Hydraulic Flow Rate Sensor2/RConn2 -- Hydraulic Constant Pressure Source/LConn1
  Hydraulic Flow Rate Sensor2/RConn3 -- PS Terminator4/LConn1
  Hydraulic Flow Rate Sensor2/RConn1 -- PS-Simulink Converter8/LConn1
  Flow meter L/s3/LConn1 -- Flow meter L/s1/RConn1 -- Flow meter L/s7/RConn1 -- Pressure Relief Valve/LConn1 -- Hydraulic Pressure Sensor1/LConn1 -- Flow meter L/s2/LConn1
  Flow meter L/s6/RConn1 -- Double-Acting Hydraulic Cylinder (Simple)/LConn2
  Check Valve4/RConn1 -- Flow meter L/s7/LConn1
  Flow meter L/s8/LConn1 -- Check Valve5/RConn1
  Subsystem/RConn1 -- Flow meter L/s3/RConn1
  Pressure Relief Valve3/LConn1 -- Subsystem/LConn1
  Flow meter L/s5/RConn1 -- Subsystem/RConn2

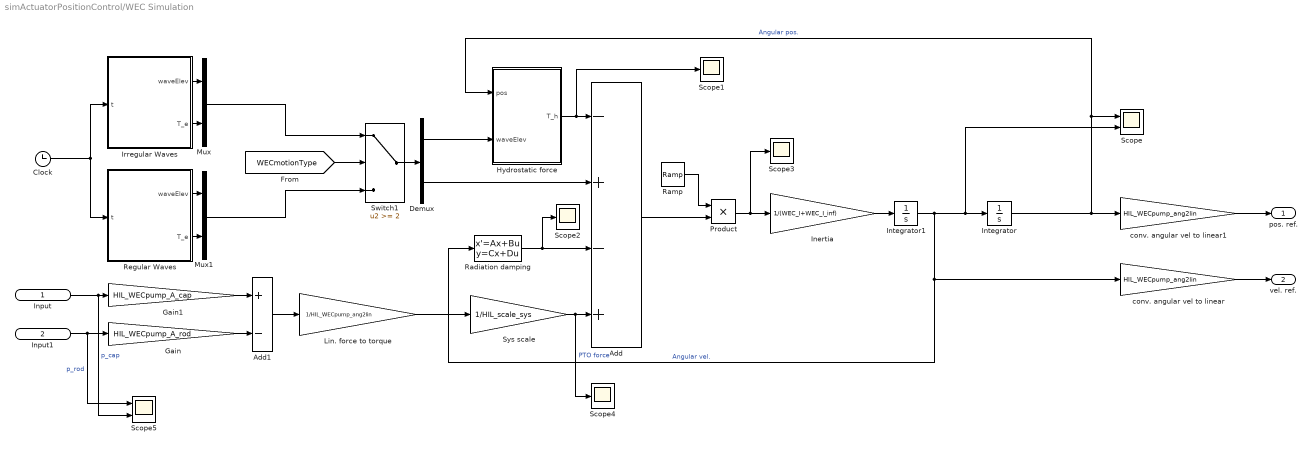
== system simActuatorPositionControl/WEC Simulation ==
  Input : Inport  SampleTime=0.01
  Input1 : Inport  Port=2  SampleTime=0.01
  Add : Sum  Inputs=-+-+
  Add1 : Sum  Inputs=+-
  Clock : Clock
  Demux : Demux  Outputs=2
  Gain : Gain  Gain=HIL_WECpump_A_rod
  Gain1 : Gain  Gain=HIL_WECpump_A_cap
  Hydrostatic force : MATLAB Function  TreatAsAtomicUnit=on
  Inertia : Gain  Gain=1/(WEC_I+WEC_I_inf)
  Integrator : Integrator
  Integrator1 : Integrator
  Irregular Waves : MATLAB Function  TreatAsAtomicUnit=on
  Lin. force to torque : Gain  Gain=1/HIL_WECpump_ang2lin
  Mux : Mux  Inputs=2
  Mux1 : Mux  Inputs=2
  Product : Product
  Radiation damping : StateSpace  A=WEC_A_rad  B=WEC_B_rad  C=[1,0,0]  D=0  InitialCondition=WEC_ICs
  Ramp : simulink/Sources/Ramp  slope=1/5  start=0.5  InitialOutput=0
  Regular Waves : MATLAB Function  TreatAsAtomicUnit=on
  Scope : Scope  NumInputPorts=2
  Scope{1..4} (4 alike) : Scope
  Scope5 : Scope  NumInputPorts=2
  Switch1 : Switch  Threshold=2  SaturateOnIntegerOverflow=off  InputSameDT=off
  Sys scale : Gain  Gain=1/HIL_scale_sys
  conv. angular vel to linear : Gain  Gain=HIL_WECpump_ang2lin
  conv. angular vel to linear1 : Gain  Gain=HIL_WECpump_ang2lin
  pos. ref. : Outport
  vel. ref. : Outport  Port=2
  wires:
  Radiation damping/1 -> Add/3, Scope2/1
  Clock/1 -> Regular Waves/1(t), Irregular Waves/1(t)
  Irregular Waves/1(waveElev) -> Mux/1
  Irregular Waves/2(T_e) -> Mux/2
  Hydrostatic force/1(T_h) -> Scope1/1, Add/1
  Inertia/1 -> Integrator1/1
  Integrator1/1 -> Scope/2, Integrator/1, Radiation damping/1, conv. angular vel to linear/1  "Angular vel."
  Integrator/1 -> conv. angular vel to linear1/1, Scope/1, Hydrostatic force/1(pos)  "Angular pos."
  Lin. force to torque/1 -> Sys scale/1
  Add1/1 -> Lin. force to torque/1
  Input/1 -> Scope5/2, Gain1/1  "p_cap"
  Input1/1 -> Scope5/1, Gain/1  "p_rod"
  conv. angular vel to linear1/1 -> pos. ref./1
  conv. angular vel to linear/1 -> vel. ref./1
  Sys scale/1 -> Scope4/1, Add/4  "PTO force"
  Gain/1 -> Add1/2
  Gain1/1 -> Add1/1
  Demux/1 -> Hydrostatic force/2(waveElev)
  [WECmotionType] -> Switch1/2
  Demux/2 -> Add/2
  Regular Waves/1(waveElev) -> Mux1/1
  Regular Waves/2(T_e) -> Mux1/2
  Switch1/1 -> Demux/1
  Mux1/1 -> Switch1/3
  Mux/1 -> Switch1/1
  Product/1 -> Scope3/1, Inertia/1
  Add/1 -> Product/2
  Ramp/1 -> Product/1

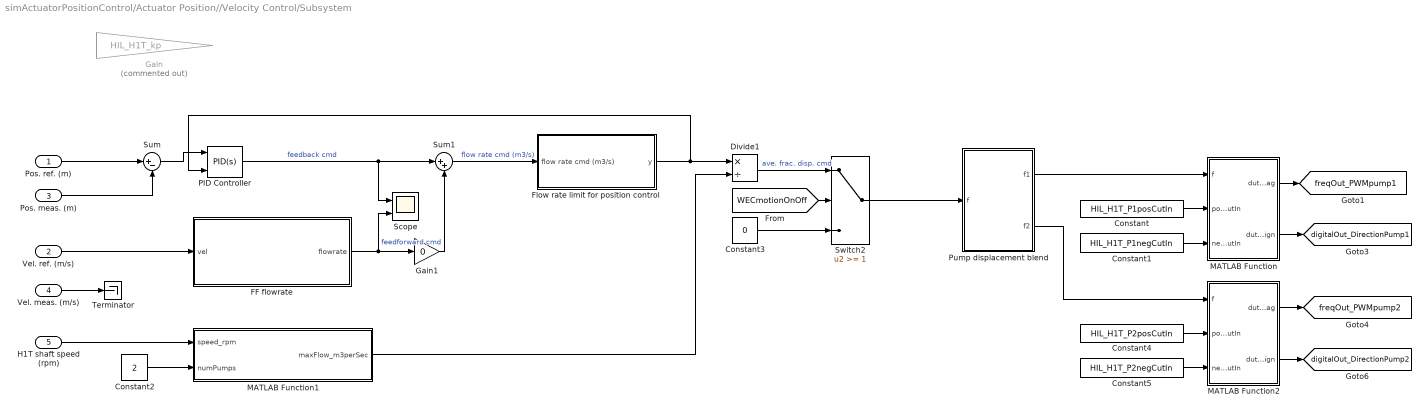
== system simActuatorPositionControl/Actuator Position//Velocity Control/Subsystem ==
  Pos. ref. (m) : Inport  SampleTime=0.01
  Vel. ref. (m/s) : Inport  Port=2  SampleTime=0.01
  Pos. meas. (m) : Inport  Port=3  SampleTime=0.01
  Vel. meas. (m/s) : Inport  Port=4  SampleTime=0.01
  H1T shaft speed (rpm) : Inport  Port=5
  Constant : Constant  Value=HIL_H1T_P1posCutIn
  Constant1 : Constant  Value=HIL_H1T_P1negCutIn
  Constant2 : Constant  Value=2
  Constant3 : Constant  Value=0
  Constant4 : Constant  Value=HIL_H1T_P2posCutIn
  Constant5 : Constant  Value=HIL_H1T_P2negCutIn
  Divide1 : Product  Inputs=*/
  FF flowrate : MATLAB Function  TreatAsAtomicUnit=on
  Flow rate limit for position control : Subsystem
  Gain : Gain  Commented=on  Gain=HIL_H1T_kp
  Gain1 : Gain  Gain=0
  MATLAB Function : MATLAB Function  TreatAsAtomicUnit=on
  MATLAB Function1 : MATLAB Function  TreatAsAtomicUnit=on
  MATLAB Function2 : MATLAB Function  TreatAsAtomicUnit=on
  PID Controller : slpidlib/PID Controller  Controller=PID  Form=Parallel  TimeDomain=Continuous-time  UseExternalTs=off  SampleTime=-1  IntegratorMethod=Forward Euler  FilterMethod=Forward Euler  ControllerParametersSource=internal  P=HIL_H1T_kp  I=HIL_H1T_ki  UseKiTs=off  D=HIL_H1T_kd  N=100  UseFilter=on  TunerSelectOption=Transfer Function Based (PID Tuner App)  InitialConditionSource=internal  InitialConditionForIntegrator=0  InitialConditionForFilter=0  DifferentiatorICPrevScaledInput=0  ExternalReset=none  TrackingMode=on  Kt=50  LimitOutput=on  SatLimitsSource=internal  UpperSaturationLimit=0.003  LowerSaturationLimit=-0.003  LinearizeAsGain=on  AntiWindupMode=none  Kb=10  POutMin=[]  POutMax=[]  IOutMin=[]  IOutMax=[]  DOutMin=[]  DOutMax=[]  NOutMin=[]  NOutMax=[]  SumOutMin=[]  SumOutMax=[]  SaturationOutMin=[]  SaturationOutMax=[]  PParamMin=[]  PParamMax=[]  IParamMin=[]  IParamMax=[]  DParamMin=[]  DParamMax=[]  NParamMin=[]  NParamMax=[]  KbParamMin=[]  KbParamMax=[]  KtParamMin=[]  KtParamMax=[]  KbOutMin=[]  KbOutMax=[]  KtOutMin=[]  KtOutMax=[]  IntegratorOutMin=[]  IntegratorOutMax=[]  FilterOutMin=[]  FilterOutMax=[]  SumI1OutMin=[]  SumI1OutMax=[]  SumI2OutMin=[]  SumI2OutMax=[]  SumI3OutMin=[]  SumI3OutMax=[]  SumI4OutMin=[]  SumI4OutMax=[]  SumDOutMin=[]  SumDOutMax=[]  DifferentiatorOutMin=[]  DifferentiatorOutMax=[]  FilterDiffOutCoefMin=[]  FilterDiffOutCoefMax=[]  ReciprocalOutMin=[]  ReciprocalOutMax=[]  SumDenOutMin=[]  SumDenOutMax=[]  SumNumOutMin=[]  SumNumOutMax=[]  DivideOutMin=[]  DivideOutMax=[]  UdiffTsProdOutMin=[]  UdiffTsProdOutMax=[]  NTsProdOutMin=[]  NTsProdOutMax=[]  UintegralTsProdOutMin=[]  UintegralTsProdOutMax=[]  UngainTsProdOutMin=[]  UngainTsProdOutMax=[]  IntegratorContinuousStateAttributes=''  IntegratorStateMustResolveToSignalObject=off  IntegratorRTWStateStorageClass=Auto  FilterContinuousStateAttributes=''  FilterStateMustResolveToSignalObject=off  FilterRTWStateStorageClass=Auto  ParallelPVariant=InternalParameters  IdealPVariant=Disabled  IVariant=InternalParameters  DVariant=InternalParameters  IntegratorVariant=Continuous  SatVariant=Enabled  AWVariant=Passthrough  PCopyVariant=Disabled  TRVariant=Enabled  FdbkBlocksVariant=Forward  IdealPFdbkVariant=Disabled  SatFdbkVariant=Disabled  DerivativeFilterVariant=ContFilter  NVariant=InternalParameters  NCopyVariant=Disabled  FilterICVariant=InternalICsFilter  IntegratorICVariant=InternalICs  ExternalResetVariant=Disabled  TRSumVariant=TrackingMode  SumFdbkVariant=Disabled  SumVariant=Sum_PID  TsampFilterVariant=InternalTs  TsampNgainVariant=Passthrough  TsampIntegralVariant=Passthrough  ExternalSaturationOutDataTypeStr=Inherit: Same as second input  aMode=0
  Pump displacement blend : MATLAB Function  TreatAsAtomicUnit=on
  Scope : Scope  NumInputPorts=2
  Sum : Sum  Inputs=|+-
  Sum1 : Sum  Inputs=|++
  Switch2 : Switch  Threshold=1  SaturateOnIntegerOverflow=off  InputSameDT=off
  Terminator : Terminator
  tag scope: digitalOut_DirectionPump1=global, digitalOut_DirectionPump2=global, freqOut_PWMpump1=global, freqOut_PWMpump2=global
  wires:
  FF flowrate/1(flowrate) -> Gain1/1, Scope/2  "feedforward cmd"
  Pos. meas. (m)/1 -> Sum/2
  MATLAB Function1/1(maxFlow_m3perSec) -> Divide1/2
  Constant2/1 -> MATLAB Function1/2(numPumps)
  Divide1/1 -> Switch2/1  "ave. frac. disp. cmd"
  H1T shaft speed (rpm)/1 -> MATLAB Function1/1(speed_rpm)
  MATLAB Function/1(dutyMag) -> [freqOut_PWMpump1]
  Constant1/1 -> MATLAB Function/3(negCutIn)
  Pos. ref. (m)/1 -> Sum/1
  Vel. ref. (m/s)/1 -> FF flowrate/1(vel)
  PID Controller/1 -> Scope/1, Sum1/1  "feedback cmd"
  MATLAB Function/2(dutySign) -> [digitalOut_DirectionPump1]
  Vel. meas. (m/s)/1 -> Terminator/1
  Sum/1 -> PID Controller/1
  Constant/1 -> MATLAB Function/2(posCutIn)
  [WECmotionOnOff] -> Switch2/2
  Constant3/1 -> Switch2/3
  Constant5/1 -> MATLAB Function2/3(negCutIn)
  MATLAB Function2/1(dutyMag) -> [freqOut_PWMpump2]
  MATLAB Function2/2(dutySign) -> [digitalOut_DirectionPump2]
  Constant4/1 -> MATLAB Function2/2(posCutIn)
  Pump displacement blend/1(f1) -> MATLAB Function/1(f)
  Pump displacement blend/2(f2) -> MATLAB Function2/1(f)
  Sum1/1 -> Flow rate limit for position control/1(flow rate cmd (m3/s))  "flow rate cmd (m3/s)"
  Flow rate limit for position control/1(y) -> PID Controller/2, Divide1/1
  Switch2/1 -> Pump displacement blend/1(f)
  Gain1/1 -> Sum1/2

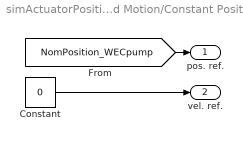
== system simActuatorPositionControl/Prescribed Motion/Constant Position ==
  Constant : Constant  Value=0
  pos. ref. : Outport
  vel. ref. : Outport  Port=2
  wires:
  [NomPosition_WECpump] -> pos. ref./1
  Constant/1 -> vel. ref./1

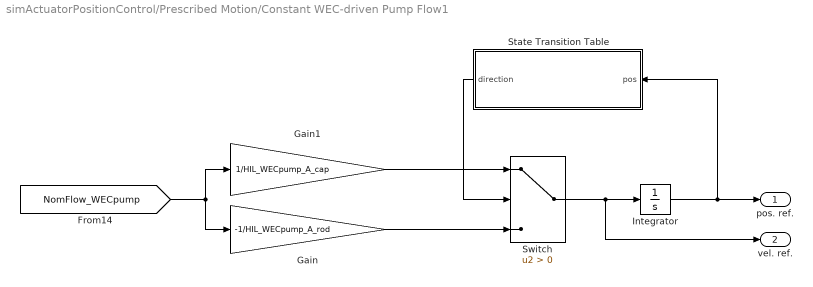
== system simActuatorPositionControl/Prescribed Motion/Constant WEC-driven Pump Flow1 ==
  Gain : Gain  Gain=-1/HIL_WECpump_A_rod
  Gain1 : Gain  Gain=1/HIL_WECpump_A_cap
  Integrator : Integrator
  State Transition Table : State Transition Table  TreatAsAtomicUnit=on
  Switch : Switch  Criteria=u2 > Threshold  SaturateOnIntegerOverflow=off  InputSameDT=off
  pos. ref. : Outport
  vel. ref. : Outport  Port=2
  wires:
  Gain1/1 -> Switch/1
  Switch/1 -> vel. ref./1, Integrator/1
  Gain/1 -> Switch/3
  [NomFlow_WECpump] -> Gain1/1, Gain/1
  Integrator/1 -> State Transition Table/1(pos), pos. ref./1
  State Transition Table/1(direction) -> Switch/2

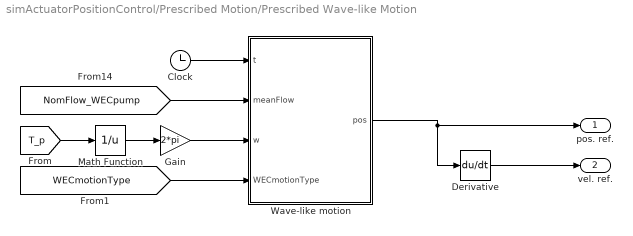
== system simActuatorPositionControl/Prescribed Motion/Prescribed Wave-like Motion ==
  Clock : Clock
  Derivative : Derivative
  Gain : Gain  Gain=2*pi
  Math Function : Math  Operator=reciprocal
  Wave-like motion : MATLAB Function  TreatAsAtomicUnit=on
  pos. ref. : Outport
  vel. ref. : Outport  Port=2
  wires:
  [NomFlow_WECpump] -> Wave-like motion/2(meanFlow)
  Wave-like motion/1(pos) -> Derivative/1, pos. ref./1
  Derivative/1 -> vel. ref./1
  Clock/1 -> Wave-like motion/1(t)
  [T_p] -> Math Function/1
  Math Function/1 -> Gain/1
  Gain/1 -> Wave-like motion/3(w)
  [WECmotionType] -> Wave-like motion/4(WECmotionType)
